simulink model "rlAgentLC"  (R2024a)
settings: Solver=VariableStepAuto  StartTime=0.0  StopTime=Tf  FixedStep=1e-3  MaxStep=0.1  RelTol=1e-3
values from neighbouring files (symbols this model uses):
  A = [ ... (first row only)    [rlAgentLCParams.m]
  B = [0 2*Cf/m 0 2*lf*Cf/Iz]'    [rlAgentLCParams.m]
  Cf = 19000    [multiAgentPFCParams.m]    (also in rlAgentLCParams.m = 151000)
  Cr = 33000    [multiAgentPFCParams.m]    (also in rlAgentLCParams.m = 146000)
  Iz = 2875    [multiAgentPFCParams.m]    (also in rlAgentLCParams.m = 1993)
  lf = 1.4    [multiAgentPFCParams.m]    (also in rlAgentLCParams.m = 1.45)
  lr = 1.6    [multiAgentPFCParams.m]    (also in rlAgentLCParams.m = 1.06)
  m = 1600    [multiAgentPFCParams.m]    (also in rlAgentLCParams.m = 1360)
  Ts = 0.1    [rlAgentLCParams.m]
  Vx = 20    [rlAgentLCParams.m]
libraries: rllib x1, matrix_library x1
settings Model: Creator=The MathWorks, Inc.  LastModifiedBy=canlab
settings SolverCC: AlgebraicLoopSolver=TrustRegion
settings DataIOCC: SaveOutput=off  SignalLogging=off  DSMLogging=off  SaveTime=off  ReturnWorkspaceOutputs=off
settings DebuggingCC: ParameterPrecisionLossMsg=none  UnconnectedInputMsg=warning  UnconnectedOutputMsg=warning  UnconnectedLineMsg=warning  ArithmeticOperatorsInVariantConditions=warning
settings ModelReferenceCC: EnableRefExpFcnMdlSchedulingChecks=on
settings SFSimCC: SimUseLocalCustomCode=off
settings RTWCC: RTWUseLocalCustomCode=off  GPUComputeCapability=3.5  DLArmComputeVersion=19.05

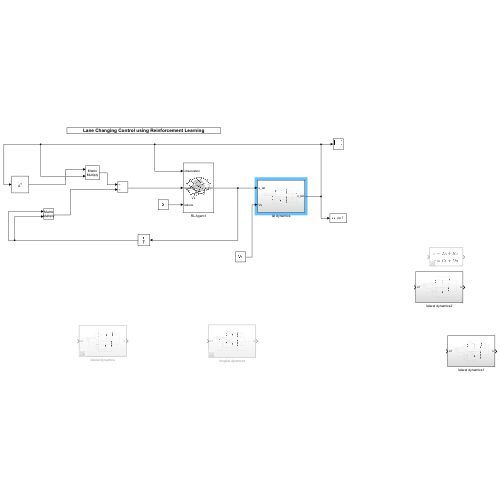
[thumbnail: Simulink's stored preview of the top-level diagram]
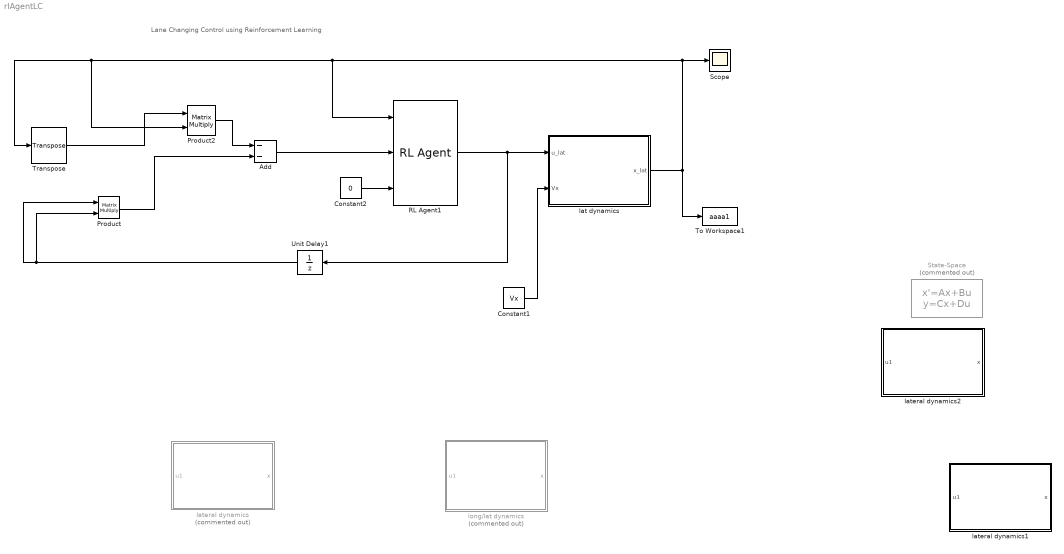
== system rlAgentLC ==
  note: Lane Changing Control using Reinforcement Learning
  Add : Sum  Inputs=--
  Constant1 : Constant  Value=Vx  SampleTime=Ts
  Constant2 : Constant  Value=0  SampleTime=Ts
  Product : Product  Multiplication=Matrix(*)
  Product2 : Product  Multiplication=Matrix(*)
  RL Agent1 : rllib/RL Agent  Agent=agent1  ExternalActionAsInput=off  ProvideLastAction=off  ProvideCumRwd=off  TreatAsDirectFeedthrough=on  UseStrictObservationDataTypes=off
  Scope : Scope
  State-Space : StateSpace  Commented=on  A=A  B=B  C=eye(4)  D=zeros(4,1)  InitialCondition=[3;0;-0.002;0]
  To Workspace1 : ToWorkspace  VariableName=aaaa1  SaveFormat=Timeseries  SampleTime=0.1
  Transpose : matrix_library/Transpose
  Unit Delay1 : UnitDelay  SampleTime=-1  HasFrameUpgradeWarning=on
  lat dynamics : Subsystem
  lateral dynamics : Subsystem  Commented=on
  lateral dynamics1 : Subsystem
  lateral dynamics2 : Subsystem
  long/lat dynamics : Subsystem  Commented=on
  wires:
  Transpose/1 -> Product2/1
  Product2/1 -> Add/1
  Constant2/1 -> RL Agent1/3
  RL Agent1/1 -> lat dynamics/1(u_lat), Unit Delay1/1
  lat dynamics/1(x_lat) -> Transpose/1, Product2/2, RL Agent1/1, Scope/1, To Workspace1/1
  Add/1 -> RL Agent1/2
  Product/1 -> Add/2
  Unit Delay1/1 -> Product/1, Product/2
  Constant1/1 -> lat dynamics/2(Vx)

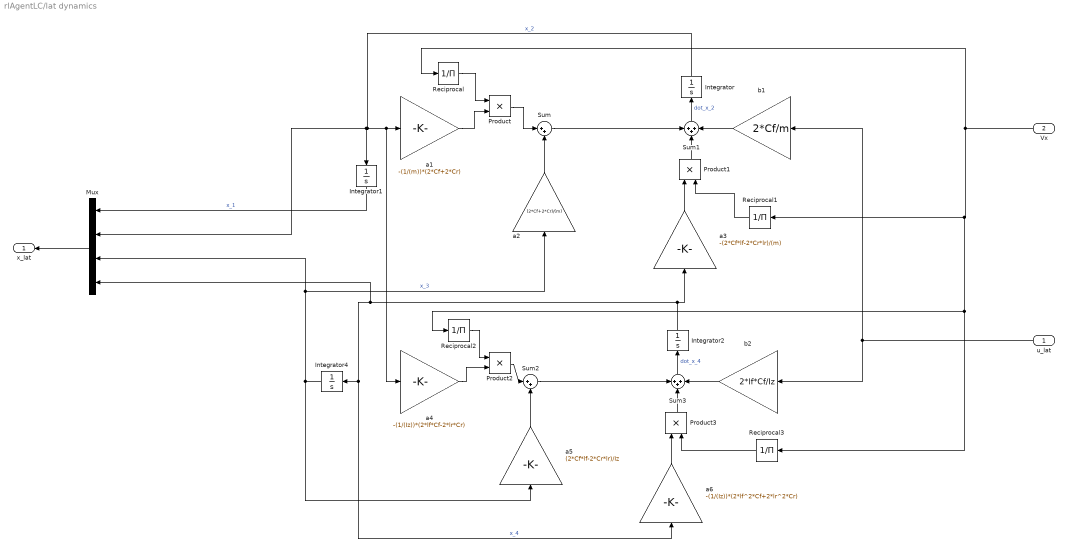
== system rlAgentLC/lat dynamics ==
  u_lat : Inport
  Vx : Inport  Port=2
  Integrator : Integrator
  Integrator1 : Integrator  InitialCondition=3
  Integrator2 : Integrator
  Integrator4 : Integrator  InitialCondition=-0.002
  Mux : Mux
  Product{,1..3} (4 alike) : Product
  Reciprocal{,1..3} (4 alike) : Product  Inputs=/
  Sum : Sum  Inputs=|++
  Sum1 : Sum  Inputs=+++
  Sum2 : Sum  Inputs=|++
  Sum3 : Sum  Inputs=+++
  a1 : Gain  Gain=-(1/(m))*(2*Cf+2*Cr)
  a2 : Gain  Gain=(2*Cf+2*Cr)/(m)
  a3 : Gain  Gain=-(2*Cf*lf-2*Cr*lr)/(m)
  a4 : Gain  Gain=-(1/(Iz))*(2*lf*Cf-2*lr*Cr)
  a5 : Gain  Gain=(2*Cf*lf-2*Cr*lr)/Iz
  a6 : Gain  Gain=-(1/(Iz))*(2*lf^2*Cf+2*lr^2*Cr)
  b1 : Gain  Gain=2*Cf/m
  b2 : Gain  Gain=2*lf*Cf/Iz
  x_lat : Outport
  wires:
  a3/1 -> Product1/1
  Product1/1 -> Sum1/2
  Sum1/1 -> Integrator/1  "dot_x_2"
  Sum3/1 -> Integrator2/1  "dot_x_4"
  Integrator1/1 -> Mux/1  "x_1"
  u_lat/1 -> b1/1, b2/1
  a2/1 -> Sum/2
  Sum2/1 -> Sum3/1
  Integrator2/1 -> a6/1, Integrator4/1, Mux/4, a3/1  "x_4"
  a4/1 -> Product2/2
  Integrator4/1 -> a2/1, Mux/3, a5/1  "x_3"
  Integrator/1 -> Mux/2, Integrator1/1, a4/1, a1/1  "x_2"
  a5/1 -> Sum2/2
  Product3/1 -> Sum3/2
  Product2/1 -> Sum2/1
  Mux/1 -> x_lat/1
  Reciprocal/1 -> Product/1
  b2/1 -> Sum3/3
  a1/1 -> Product/2
  Vx/1 -> Reciprocal2/1, Reciprocal3/1, Reciprocal1/1, Reciprocal/1
  Reciprocal2/1 -> Product2/1
  Reciprocal1/1 -> Product1/2
  Product/1 -> Sum/1
  Sum/1 -> Sum1/1
  b1/1 -> Sum1/3
  a6/1 -> Product3/1
  Reciprocal3/1 -> Product3/2

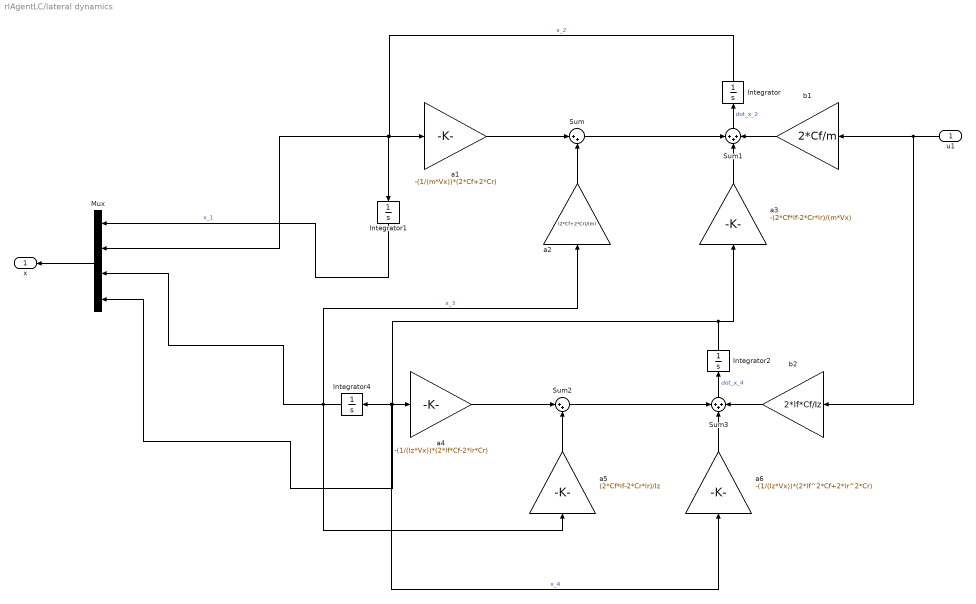
== system rlAgentLC/lateral dynamics ==
  u1 : Inport
  Integrator : Integrator
  Integrator1 : Integrator  InitialCondition=1
  Integrator2 : Integrator
  Integrator4 : Integrator  InitialCondition=1
  Mux : Mux
  Sum : Sum  Inputs=|++
  Sum1 : Sum  Inputs=+++
  Sum2 : Sum  Inputs=|++
  Sum3 : Sum  Inputs=+++
  a1 : Gain  Gain=-(1/(m*Vx))*(2*Cf+2*Cr)
  a2 : Gain  Gain=(2*Cf+2*Cr)/(m)
  a3 : Gain  Gain=-(2*Cf*lf-2*Cr*lr)/(m*Vx)
  a4 : Gain  Gain=-(1/(Iz*Vx))*(2*lf*Cf-2*lr*Cr)
  a5 : Gain  Gain=(2*Cf*lf-2*Cr*lr)/Iz
  a6 : Gain  Gain=-(1/(Iz*Vx))*(2*lf^2*Cf+2*lr^2*Cr)
  b1 : Gain  Gain=2*Cf/m
  b2 : Gain  Gain=2*lf*Cf/Iz
  x : Outport
  wires:
  Integrator/1 -> Mux/2, Integrator1/1, a1/1  "x_2"
  a6/1 -> Sum3/2
  Sum/1 -> Sum1/1
  a4/1 -> Sum2/1
  Integrator4/1 -> a5/1, a2/1, Mux/3  "x_3"
  a5/1 -> Sum2/2
  Integrator2/1 -> a6/1, Integrator4/1, a4/1, Mux/4, a3/1  "x_4"
  Sum1/1 -> Integrator/1  "dot_x_2"
  Sum2/1 -> Sum3/1
  Sum3/1 -> Integrator2/1  "dot_x_4"
  b2/1 -> Sum3/3
  b1/1 -> Sum1/3
  a2/1 -> Sum/2
  a3/1 -> Sum1/2
  a1/1 -> Sum/1
  u1/1 -> b2/1, b1/1
  Integrator1/1 -> Mux/1  "x_1"
  Mux/1 -> x/1

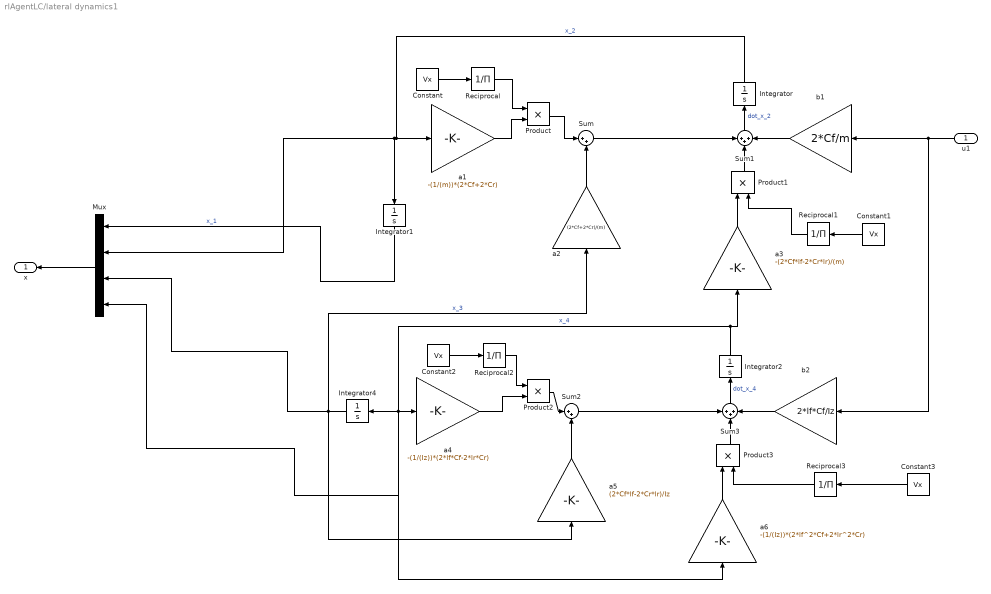
== system rlAgentLC/lateral dynamics1 ==
  u1 : Inport
  Constant{,1..3} (4 alike) : Constant  Value=Vx
  Integrator : Integrator
  Integrator1 : Integrator  InitialCondition=3
  Integrator2 : Integrator
  Integrator4 : Integrator  InitialCondition=-0.002
  Mux : Mux
  Product{,1..3} (4 alike) : Product
  Reciprocal{,1..3} (4 alike) : Product  Inputs=/
  Sum : Sum  Inputs=|++
  Sum1 : Sum  Inputs=+++
  Sum2 : Sum  Inputs=|++
  Sum3 : Sum  Inputs=+++
  a1 : Gain  Gain=-(1/(m))*(2*Cf+2*Cr)
  a2 : Gain  Gain=(2*Cf+2*Cr)/(m)
  a3 : Gain  Gain=-(2*Cf*lf-2*Cr*lr)/(m)
  a4 : Gain  Gain=-(1/(Iz))*(2*lf*Cf-2*lr*Cr)
  a5 : Gain  Gain=(2*Cf*lf-2*Cr*lr)/Iz
  a6 : Gain  Gain=-(1/(Iz))*(2*lf^2*Cf+2*lr^2*Cr)
  b1 : Gain  Gain=2*Cf/m
  b2 : Gain  Gain=2*lf*Cf/Iz
  x : Outport
  wires:
  Integrator/1 -> Mux/2, Integrator1/1, a1/1  "x_2"
  a6/1 -> Product3/1
  Sum/1 -> Sum1/1
  a4/1 -> Product2/2
  Integrator4/1 -> a5/1, a2/1, Mux/3  "x_3"
  a5/1 -> Sum2/2
  Integrator2/1 -> a6/1, Integrator4/1, a4/1, Mux/4, a3/1  "x_4"
  Sum1/1 -> Integrator/1  "dot_x_2"
  Sum2/1 -> Sum3/1
  Sum3/1 -> Integrator2/1  "dot_x_4"
  b2/1 -> Sum3/3
  b1/1 -> Sum1/3
  a2/1 -> Sum/2
  a3/1 -> Product1/1
  a1/1 -> Product/2
  u1/1 -> b2/1, b1/1
  Integrator1/1 -> Mux/1  "x_1"
  Mux/1 -> x/1
  Reciprocal/1 -> Product/1
  Constant/1 -> Reciprocal/1
  Product/1 -> Sum/1
  Constant1/1 -> Reciprocal1/1
  Reciprocal1/1 -> Product1/2
  Product1/1 -> Sum1/2
  Constant2/1 -> Reciprocal2/1
  Reciprocal2/1 -> Product2/1
  Product2/1 -> Sum2/1
  Constant3/1 -> Reciprocal3/1
  Reciprocal3/1 -> Product3/2
  Product3/1 -> Sum3/2

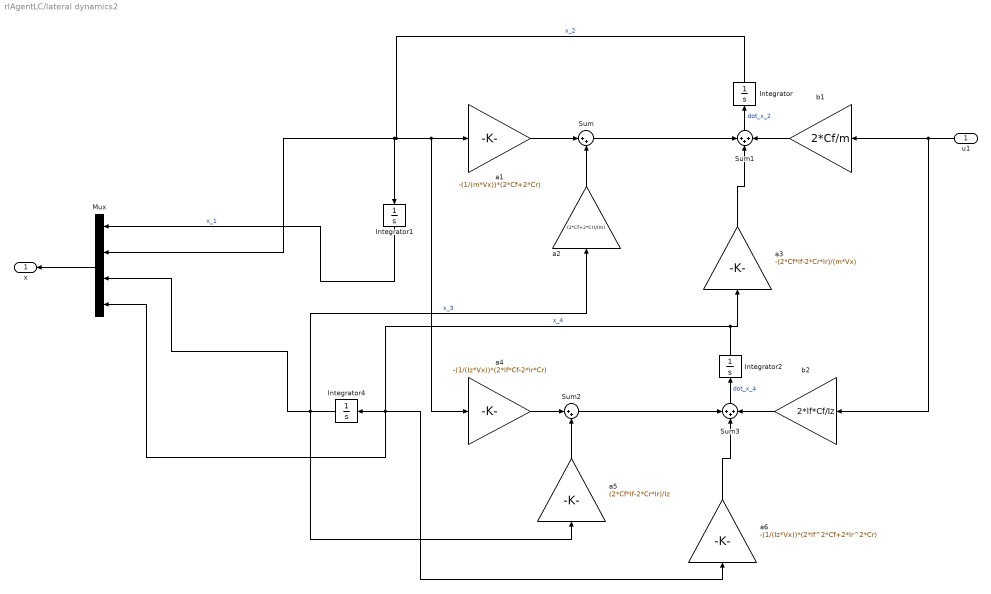
== system rlAgentLC/lateral dynamics2 ==
  u1 : Inport
  Integrator : Integrator
  Integrator1 : Integrator  InitialCondition=3
  Integrator2 : Integrator
  Integrator4 : Integrator  InitialCondition=-0.002
  Mux : Mux
  Sum : Sum  Inputs=|++
  Sum1 : Sum  Inputs=+++
  Sum2 : Sum  Inputs=|++
  Sum3 : Sum  Inputs=+++
  a1 : Gain  Gain=-(1/(m*Vx))*(2*Cf+2*Cr)
  a2 : Gain  Gain=(2*Cf+2*Cr)/(m)
  a3 : Gain  Gain=-(2*Cf*lf-2*Cr*lr)/(m*Vx)
  a4 : Gain  Gain=-(1/(Iz*Vx))*(2*lf*Cf-2*lr*Cr)
  a5 : Gain  Gain=(2*Cf*lf-2*Cr*lr)/Iz
  a6 : Gain  Gain=-(1/(Iz*Vx))*(2*lf^2*Cf+2*lr^2*Cr)
  b1 : Gain  Gain=2*Cf/m
  b2 : Gain  Gain=2*lf*Cf/Iz
  x : Outport
  wires:
  Integrator/1 -> Mux/2, Integrator1/1, a1/1, a4/1  "x_2"
  Sum/1 -> Sum1/1
  Integrator4/1 -> a5/1, a2/1, Mux/3  "x_3"
  a5/1 -> Sum2/2
  Integrator2/1 -> a6/1, Integrator4/1, Mux/4, a3/1  "x_4"
  Sum1/1 -> Integrator/1  "dot_x_2"
  Sum2/1 -> Sum3/1
  Sum3/1 -> Integrator2/1  "dot_x_4"
  b2/1 -> Sum3/3
  b1/1 -> Sum1/3
  a2/1 -> Sum/2
  u1/1 -> b2/1, b1/1
  Integrator1/1 -> Mux/1  "x_1"
  Mux/1 -> x/1
  a1/1 -> Sum/1
  a3/1 -> Sum1/2
  a4/1 -> Sum2/1
  a6/1 -> Sum3/2

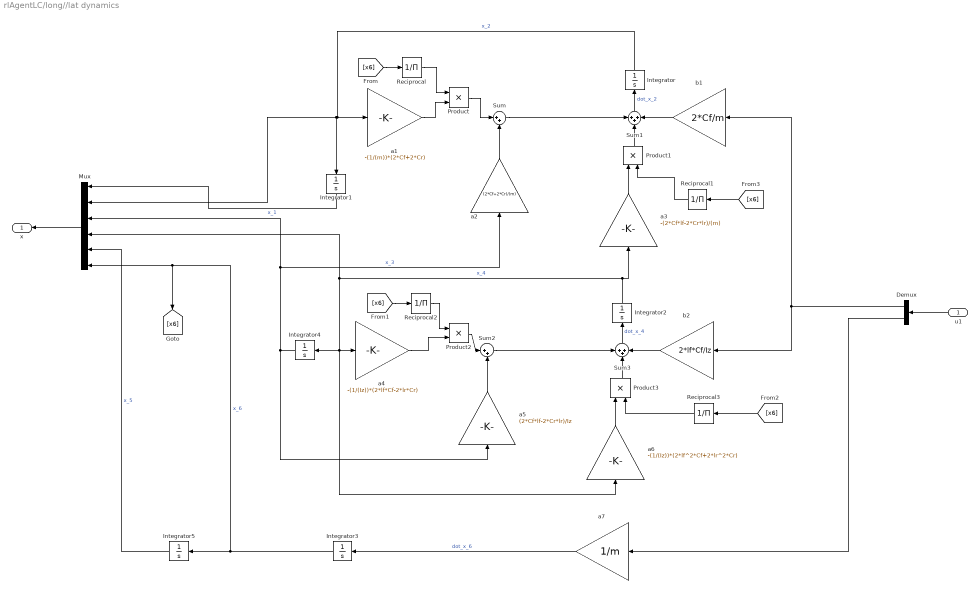
== system rlAgentLC/long//lat dynamics ==
  u1 : Inport
  Demux : Demux  Outputs=2
  Integrator : Integrator
  Integrator{1,3..5} (4 alike) : Integrator  InitialCondition=1
  Integrator2 : Integrator
  Mux : Mux  Inputs=6
  Product{,1..3} (4 alike) : Product
  Reciprocal{,1..3} (4 alike) : Product  Inputs=/
  Sum : Sum  Inputs=|++
  Sum1 : Sum  Inputs=+++
  Sum2 : Sum  Inputs=|++
  Sum3 : Sum  Inputs=+++
  a1 : Gain  Gain=-(1/(m))*(2*Cf+2*Cr)
  a2 : Gain  Gain=(2*Cf+2*Cr)/(m)
  a3 : Gain  Gain=-(2*Cf*lf-2*Cr*lr)/(m)
  a4 : Gain  Gain=-(1/(Iz))*(2*lf*Cf-2*lr*Cr)
  a5 : Gain  Gain=(2*Cf*lf-2*Cr*lr)/Iz
  a6 : Gain  Gain=-(1/(Iz))*(2*lf^2*Cf+2*lr^2*Cr)
  a7 : Gain  Gain=1/m
  b1 : Gain  Gain=2*Cf/m
  b2 : Gain  Gain=2*lf*Cf/Iz
  x : Outport
  wires:
  Demux/2 -> a7/1
  a7/1 -> Integrator3/1  "dot_x_6"
  Integrator3/1 -> [x6], Mux/6, Integrator5/1  "x_6"
  Integrator5/1 -> Mux/5  "x_5"
  a3/1 -> Product1/1
  Product1/1 -> Sum1/2
  Sum1/1 -> Integrator/1  "dot_x_2"
  Sum3/1 -> Integrator2/1  "dot_x_4"
  Integrator1/1 -> Mux/1  "x_1"
  Demux/1 -> b1/1, b2/1
  a2/1 -> Sum/2
  Sum2/1 -> Sum3/1
  Integrator2/1 -> a6/1, Integrator4/1, a4/1, Mux/4, a3/1  "x_4"
  a4/1 -> Product2/2
  Integrator4/1 -> a2/1, Mux/3, a5/1  "x_3"
  Integrator/1 -> Mux/2, Integrator1/1, a1/1  "x_2"
  a5/1 -> Sum2/2
  Product3/1 -> Sum3/2
  Product2/1 -> Sum2/1
  [x6] -> Reciprocal1/1
  [x6] -> Reciprocal3/1
  Mux/1 -> x/1
  Reciprocal/1 -> Product/1
  b2/1 -> Sum3/3
  a1/1 -> Product/2
  [x6] -> Reciprocal2/1
  Reciprocal2/1 -> Product2/1
  Reciprocal1/1 -> Product1/2
  Product/1 -> Sum/1
  Sum/1 -> Sum1/1
  b1/1 -> Sum1/3
  a6/1 -> Product3/1
  Reciprocal3/1 -> Product3/2
  [x6] -> Reciprocal/1
  u1/1 -> Demux/1
